simulink model "AFS_DD1ms"  (R2016b)
settings: configuration reference "CodeGenConfigSet" (kept outside this file)
values from neighbouring files (symbols this model uses):
  AFS_dmTransf_CUR = Calibration.Parameter    [init_AFS_DD1ms.m]    (also in init_AFS_DD1ms_SIL.m = Simulink.Parameter)
  AFS_dmTransf_CURX = Calibration.Parameter    [init_AFS_DD1ms.m]    (also in init_AFS_DD1ms_SIL.m = Simulink.Parameter)
  AFS_numSmplMax_C = Calibration.Parameter    [init_AFS_DD1ms.m]    (also in init_AFS_DD1ms_SIL.m = Simulink.Parameter)
undefined symbols (not defined in the file or in its folder): EpmSynState_conv
libraries: simulink x1
settings Model: Creator=Colin  LastModifiedBy=liutao
settings ConfigSetRef: SourceLocation=Base Workspace

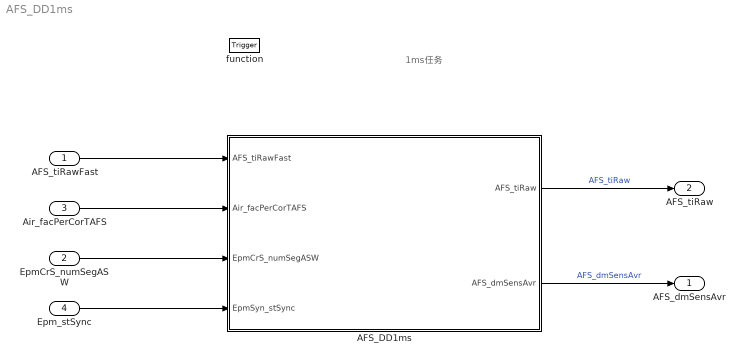
== system AFS_DD1ms ==
  note: 1ms任务
  AFS_tiRawFast : Inport  Tag=us  Description=Raw air mass period  OutMin=0  OutMax=107374182  OutDataTypeStr=Time_PwmHigh_us
  EpmCrS_numSegASW : Inport  Description=counter of part segments  Port=2  OutMin=0  OutMax=255  OutDataTypeStr=State_uint8
  Air_facPerCorTAFS : Inport  Description=Period correction factor for air mass signal.  Port=3  OutMin=-4  OutMax=3.9999  OutDataTypeStr=Fact8192
  Epm_stSync : Inport  Description=State of synchronization  Port=4  OutDataTypeStr=Enum: EpmSynState_conv
  function : TriggerPort  TriggerType=function-call  VariantControl=Variant
  AFS_DD1ms : Subsystem
  AFS_dmSensAvr : Outport  Tag=kg/h  Description=Averaged Sensed air mass flow  OutMin=-8192  OutMax=8191  OutDataTypeStr=AirMassPerTime
  AFS_tiRaw : Outport  Tag=us  Description=Raw air mass period  Port=2  OutMin=0  OutMax=107374182  OutDataTypeStr=Time_PwmHigh_us
  wires:
  EpmCrS_numSegASW/1 -> AFS_DD1ms/3(EpmCrS_numSegASW)
  AFS_tiRawFast/1 -> AFS_DD1ms/1(AFS_tiRawFast)
  AFS_DD1ms/1(AFS_tiRaw) -> AFS_tiRaw/1  "AFS_tiRaw"
  AFS_DD1ms/2(AFS_dmSensAvr) -> AFS_dmSensAvr/1  "AFS_dmSensAvr"
  Air_facPerCorTAFS/1 -> AFS_DD1ms/2(Air_facPerCorTAFS)
  Epm_stSync/1 -> AFS_DD1ms/4(EpmSyn_stSync)

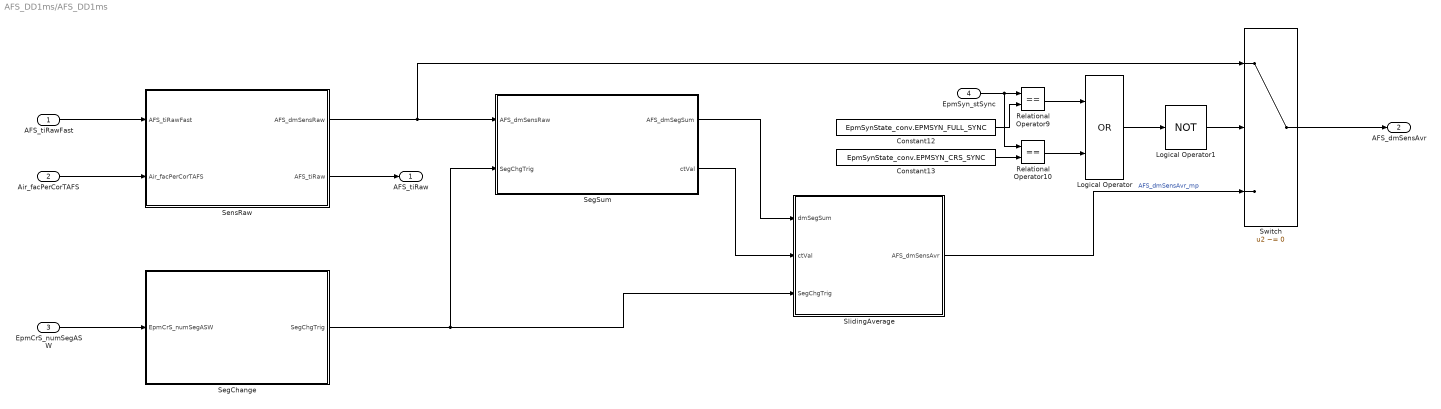
== system AFS_DD1ms/AFS_DD1ms ==
  AFS_tiRawFast : Inport
  Air_facPerCorTAFS : Inport  Port=2  OutDataTypeStr=Fact8192
  EpmCrS_numSegASW : Inport  Port=3
  EpmSyn_stSync : Inport  Port=4
  Constant12 : Constant  Value=EpmSynState_conv.EPMSYN_FULL_SYNC
  Constant13 : Constant  Value=EpmSynState_conv.EPMSYN_CRS_SYNC
  Logical Operator : Logic  Operator=OR  AllPortsSameDT=off  OutDataTypeStr=boolean
  Logical Operator1 : Logic  Operator=NOT  AllPortsSameDT=off  OutDataTypeStr=boolean
  Relational Operator10 : RelationalOperator  Operator===  OutDataTypeStr=boolean  RndMeth=Simplest
  Relational Operator9 : RelationalOperator  Operator===  OutDataTypeStr=boolean  RndMeth=Simplest
  SegChange : Subsystem
  SegSum : Subsystem
  SensRaw : Subsystem
  SlidingAverage : Subsystem
  Switch : Switch  Criteria=u2 ~= 0
  AFS_tiRaw : Outport
  AFS_dmSensAvr : Outport  Port=2
  wires:
  EpmCrS_numSegASW/1 -> SegChange/1(EpmCrS_numSegASW)
  SensRaw/2(AFS_tiRaw) -> AFS_tiRaw/1
  AFS_tiRawFast/1 -> SensRaw/1(AFS_tiRawFast)
  SensRaw/1(AFS_dmSensRaw) -> Switch/1, SegSum/1(AFS_dmSensRaw)
  SegSum/2(ctVal) -> SlidingAverage/2(ctVal)
  SegSum/1(AFS_dmSegSum) -> SlidingAverage/1(dmSegSum)
  Air_facPerCorTAFS/1 -> SensRaw/2(Air_facPerCorTAFS)
  SegChange/1(SegChgTrig) -> SlidingAverage/3(SegChgTrig), SegSum/2(SegChgTrig)
  EpmSyn_stSync/1 -> Relational Operator10/1, Relational Operator9/1
  Constant12/1 -> Relational Operator9/2
  Constant13/1 -> Relational Operator10/2
  Relational Operator9/1 -> Logical Operator/1
  Relational Operator10/1 -> Logical Operator/2
  Logical Operator/1 -> Logical Operator1/1
  Logical Operator1/1 -> Switch/2
  SlidingAverage/1(AFS_dmSensAvr) -> Switch/3  "AFS_dmSensAvr_mp"
  Switch/1 -> AFS_dmSensAvr/1

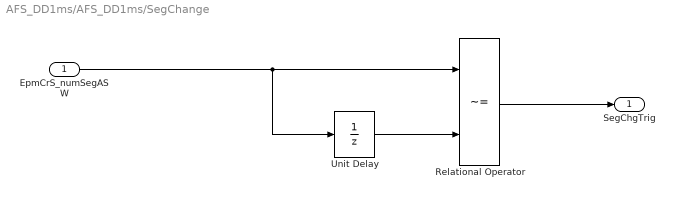
== system AFS_DD1ms/AFS_DD1ms/SegChange ==
  EpmCrS_numSegASW : Inport
  Relational Operator : RelationalOperator  Operator=~=  OutDataTypeStr=boolean  RndMeth=Simplest
  Unit Delay : UnitDelay  SampleTime=-1
      settings: AttributesFormatString=InitialValue=%<InitialCondition>
  SegChgTrig : Outport
  wires:
  EpmCrS_numSegASW/1 -> Unit Delay/1, Relational Operator/1
  Unit Delay/1 -> Relational Operator/2
  Relational Operator/1 -> SegChgTrig/1

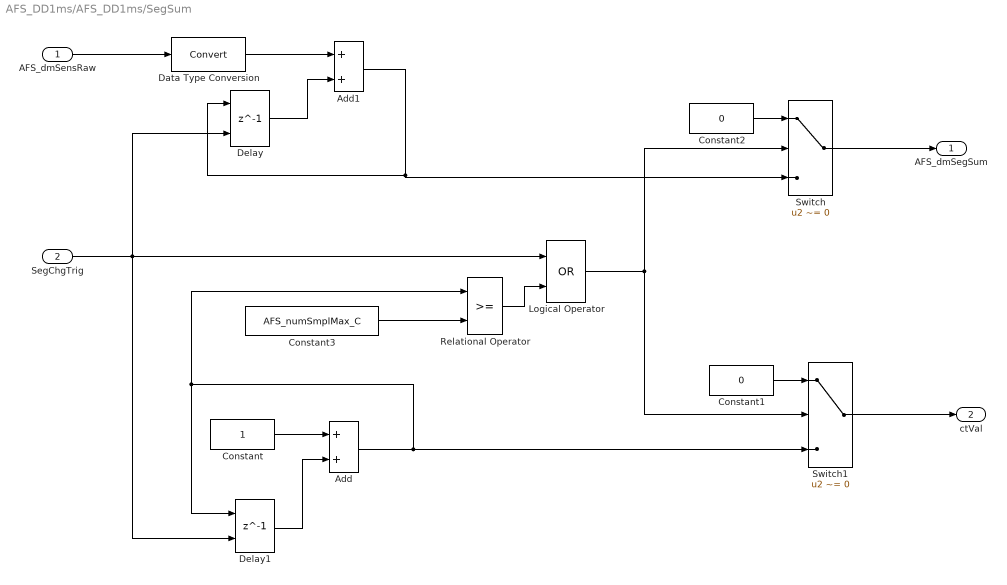
== system AFS_DD1ms/AFS_DD1ms/SegSum ==
  AFS_dmSensRaw : Inport
  SegChgTrig : Inport  Port=2
  Add : Sum
  Add1 : Sum  AccumDataTypeStr=fixdt(1,32,0.25,0)  SaturateOnIntegerOverflow=on
  Constant : Constant  OutDataTypeStr=State_uint8
  Constant1 : Constant  Value=0  OutDataTypeStr=State_uint8
  Constant2 : Constant  Value=0  OutDataTypeStr=AirMassPerTime
  Constant3 : Constant  Value=AFS_numSmplMax_C
  Data Type Conversion : DataTypeConversion
  Delay : Delay  DelayLength=1  InitialCondition=0  ExternalReset=Falling
      settings: InputPortMap=u0,r5
  Delay1 : Delay  DelayLength=1  InitialCondition=0  ExternalReset=Falling
      settings: InputPortMap=u0,r5
  Logical Operator : Logic  Operator=OR  AllPortsSameDT=off  OutDataTypeStr=boolean
  Relational Operator : RelationalOperator  OutDataTypeStr=boolean  RndMeth=Simplest  InputSameDT=on
  Switch : Switch  Criteria=u2 ~= 0
  Switch1 : Switch  Criteria=u2 ~= 0
  AFS_dmSegSum : Outport  OutDataTypeStr=fixdt(1,32,0.25,0)
  ctVal : Outport  Port=2
  wires:
  Add/1 -> Switch1/3, Relational Operator/1, Delay1/1
  Constant/1 -> Add/1
  Add1/1 -> Delay/1, Switch/3
  AFS_dmSensRaw/1 -> Data Type Conversion/1
  SegChgTrig/1 -> Delay1/2, Logical Operator/1, Delay/2
  Switch/1 -> AFS_dmSegSum/1
  Switch1/1 -> ctVal/1
  Constant1/1 -> Switch1/1
  Constant2/1 -> Switch/1
  Delay/1 -> Add1/2
  Delay1/1 -> Add/2
  Logical Operator/1 -> Switch1/2, Switch/2
  Relational Operator/1 -> Logical Operator/2
  Constant3/1 -> Relational Operator/2
  Data Type Conversion/1 -> Add1/1

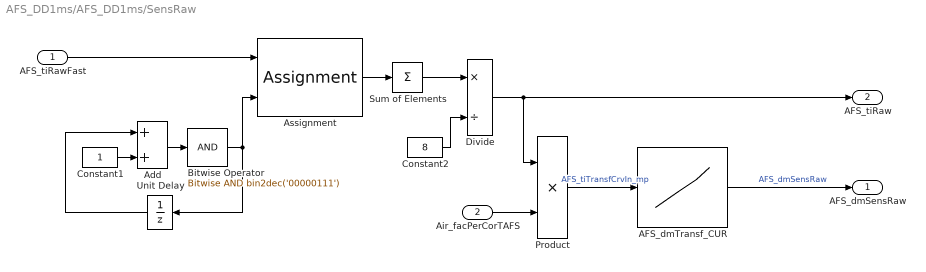
== system AFS_DD1ms/AFS_DD1ms/SensRaw ==
  AFS_tiRawFast : Inport
  Air_facPerCorTAFS : Inport  Port=2
  AFS_dmTransf_CUR : Lookup_n-D  NumberOfTableDimensions=1  BreakpointsForDimension1=AFS_dmTransf_CURX  Table=AFS_dmTransf_CUR  TableDataTypeStr=Inherit: Inherit from 'Table data'  ExtrapMethod=Clip  InternalRulePriority=Speed  OutDataTypeStr=Inherit: Inherit from 'Table data'  RndMeth=Simplest  InputSameDT=on
  Add : Sum  OutDataTypeStr=uint8
  Assignment : Assignment  IndexMode=Zero-based  OutputInitialize=Specify size for each dimension in table  DiagnosticForDimensions=Warning  IndexOptions=Index vector (port)  Indices=1  OutputSizes=8
  Bitwise Operator : simulink/Logic and Bit Operations/Bitwise Operator  logicop=AND  UseBitMask=on  BitMask=bin2dec('00000111')  BitMaskRealWorld=Stored Integer
  Constant1 : Constant  OutDataTypeStr=uint8
  Constant2 : Constant  Value=8  OutDataTypeStr=uint8
  Divide : Product  Inputs=*/  OutDataTypeStr=Inherit: Same as first input
  Product : Product  OutDataTypeStr=Inherit: Inherit via back propagation  SaturateOnIntegerOverflow=on
  Sum of Elements : Sum  Inputs=+
  Unit Delay : UnitDelay  SampleTime=-1
  AFS_dmSensRaw : Outport  OutputWhenDisabled=reset  InitialOutput=0
  AFS_tiRaw : Outport  Port=2
  wires:
  Product/1 -> AFS_dmTransf_CUR/1  "AFS_tiTransfCrvIn_mp"
  AFS_dmTransf_CUR/1 -> AFS_dmSensRaw/1  "AFS_dmSensRaw"
  Air_facPerCorTAFS/1 -> Product/2
  Assignment/1 -> Sum of Elements/1
  Add/1 -> Bitwise Operator/1
  Constant1/1 -> Add/2
  Bitwise Operator/1 -> Assignment/2, Unit Delay/1
  Unit Delay/1 -> Add/1
  Sum of Elements/1 -> Divide/1
  Divide/1 -> Product/1, AFS_tiRaw/1
  Constant2/1 -> Divide/2
  AFS_tiRawFast/1 -> Assignment/1

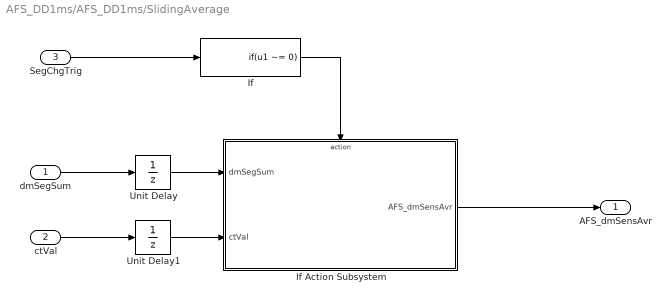
== system AFS_DD1ms/AFS_DD1ms/SlidingAverage ==
  dmSegSum : Inport
  ctVal : Inport  Port=2
  SegChgTrig : Inport  Port=3
  If : If  IfExpression=u1 ~= 0  ShowElse=off
  If Action Subsystem : Subsystem  TreatAsAtomicUnit=on
  Unit Delay : UnitDelay  SampleTime=-1
      settings: AttributesFormatString=InitialValue=%<InitialCondition>
  Unit Delay1 : UnitDelay  SampleTime=-1
      settings: AttributesFormatString=InitialValue=%<InitialCondition>
  AFS_dmSensAvr : Outport
  wires:
  If Action Subsystem/1(AFS_dmSensAvr) -> AFS_dmSensAvr/1
  SegChgTrig/1 -> If/1
  If/1 -> If Action Subsystem/Action
  dmSegSum/1 -> Unit Delay/1
  ctVal/1 -> Unit Delay1/1
  Unit Delay/1 -> If Action Subsystem/1(dmSegSum)
  Unit Delay1/1 -> If Action Subsystem/2(ctVal)

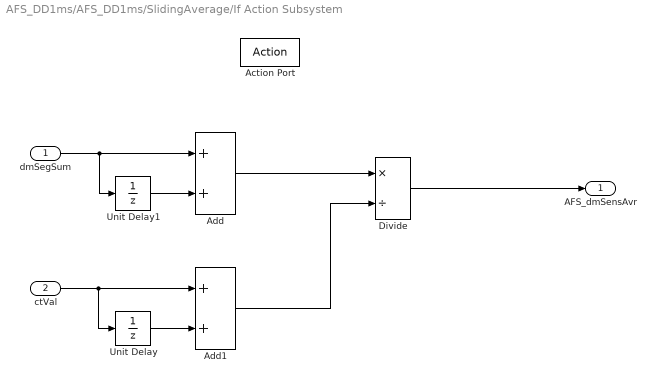
== system AFS_DD1ms/AFS_DD1ms/SlidingAverage/If Action Subsystem ==
  dmSegSum : Inport
  ctVal : Inport  Port=2
  Action Port : ActionPort  ActionType=then
  Add : Sum  SaturateOnIntegerOverflow=on
  Add1 : Sum  SaturateOnIntegerOverflow=on
  Divide : Product  Inputs=*/  OutDataTypeStr=Inherit: Inherit via back propagation  SaturateOnIntegerOverflow=on
  Unit Delay : UnitDelay  SampleTime=-1
      settings: AttributesFormatString=InitialValue=%<InitialCondition>
  Unit Delay1 : UnitDelay  SampleTime=-1
      settings: AttributesFormatString=InitialValue=%<InitialCondition>
  AFS_dmSensAvr : Outport
  wires:
  ctVal/1 -> Unit Delay/1, Add1/1
  Add1/1 -> Divide/2
  Add/1 -> Divide/1
  dmSegSum/1 -> Unit Delay1/1, Add/1
  Divide/1 -> AFS_dmSensAvr/1
  Unit Delay1/1 -> Add/2
  Unit Delay/1 -> Add1/2
